simulink model "showSampleTimes"  (R2024b)
settings: Solver=VariableStepAuto  StartTime=0.0  StopTime=10.0  RelTol=1e-3
settings Model: Creator=grouleau  LastModifiedBy=grouleau

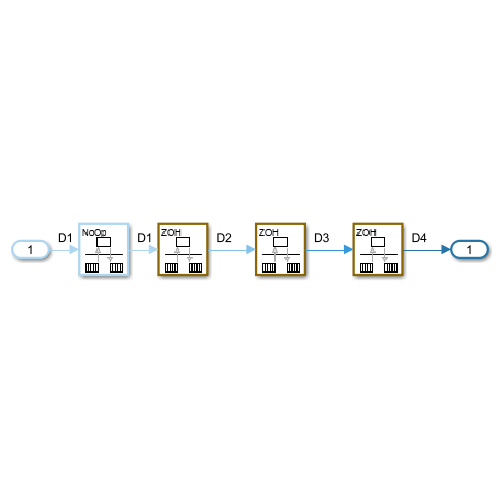
[thumbnail: Simulink's stored preview of the top-level diagram]
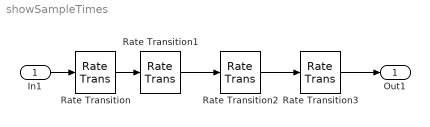
== system showSampleTimes ==
  In1 : Inport
  Rate Transition : RateTransition  OutPortSampleTime=0.01
  Rate Transition1 : RateTransition  OutPortSampleTime=0.1
  Rate Transition2 : RateTransition  OutPortSampleTime=0.2
  Rate Transition3 : RateTransition  OutPortSampleTime=1
  Out1 : Outport
  wires:
  In1/1 -> Rate Transition/1
  Rate Transition/1 -> Rate Transition1/1
  Rate Transition1/1 -> Rate Transition2/1
  Rate Transition2/1 -> Rate Transition3/1
  Rate Transition3/1 -> Out1/1
